simulink model "NeuronSizeActivity"  (Simulink 9.2)
settings: Solver=ode45  StartTime=0.0  StopTime=1  MaxStep=0.001  RelTol=1e-3  EnableMultiTasking=on
libraries: NeuroModelerLibrary x56
settings Model: Creator=Timba  LastModifiedBy=Bakhshiev  ExtModeTrigMode=oneshot  ExtModeArmWhenConnect=off
settings DataIOCC: LimitDataPoints=off
settings OptimizationCC: BlockReduction=off  BooleanDataType=off
settings DebuggingCC: SaveWithParameterizedLinksMsg=none  SignalResolutionControl=TryResolveAllWithWarning  MultiTaskDSMMsg=warning  MultiTaskCondExecSysMsg=none  FcnCallInpInsideContextMsg=error  StateNameClashWarn=none
settings HardwareCC: TargetUnknown=on
settings GRTTargetCC: TargetFcnLib=ansi_tfl_tmw.mat
settings ConfigComp: CovSFcnEnable=off

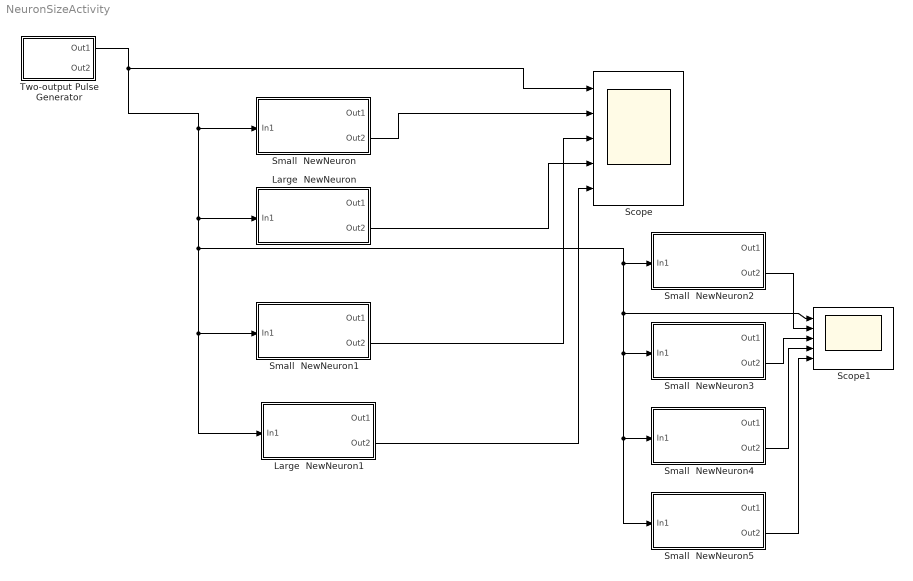
== system NeuronSizeActivity ==
  Large  NewNeuron : Subsystem
  Large  NewNeuron1 : Subsystem
  Scope : Scope  NumInputPorts=5
  Scope1 : Scope  NumInputPorts=5
  Small  NewNeuron : Subsystem
  Small  NewNeuron1 : Subsystem
  Small  NewNeuron2 : Subsystem
  Small  NewNeuron3 : Subsystem
  Small  NewNeuron4 : Subsystem
  Small  NewNeuron5 : Subsystem
  Two-output Pulse Generator : Subsystem  mask{A=100, P1=400, P2=100, PW=1, ST=0.001, OOn1=0.04, OOff1=0.5, OOn2=0.4, OOff2=20}
      mask prompts: A "Amplitude"; P1 "Out1: Period (number of samples)"; P2 "Out2: Period (number of samples)"; PW "Pulse Width (number of samples)"; ST "Sample Time"; OOn1 "Out1 On (seconds)"; OOff1 "Out1 Off (seconds)"; OOn2 "Out2 On (seconds)"; OOff2 "Out2 Off (seconds)"
  wires:
  Two-output Pulse Generator/1(Out1) -> Small  NewNeuron/1(In1), Large  NewNeuron/1(In1), Small  NewNeuron1/1(In1), Large  NewNeuron1/1(In1), Small  NewNeuron2/1(In1), Small  NewNeuron3/1(In1), Small  NewNeuron4/1(In1), Small  NewNeuron5/1(In1), Scope1/1, Scope/1
  Small  NewNeuron/2(Out2) -> Scope/2
  Small  NewNeuron1/2(Out2) -> Scope/3
  Large  NewNeuron1/2(Out2) -> Scope/5
  Large  NewNeuron/2(Out2) -> Scope/4
  Small  NewNeuron2/2(Out2) -> Scope1/2
  Small  NewNeuron3/2(Out2) -> Scope1/3
  Small  NewNeuron4/2(Out2) -> Scope1/4
  Small  NewNeuron5/2(Out2) -> Scope1/5

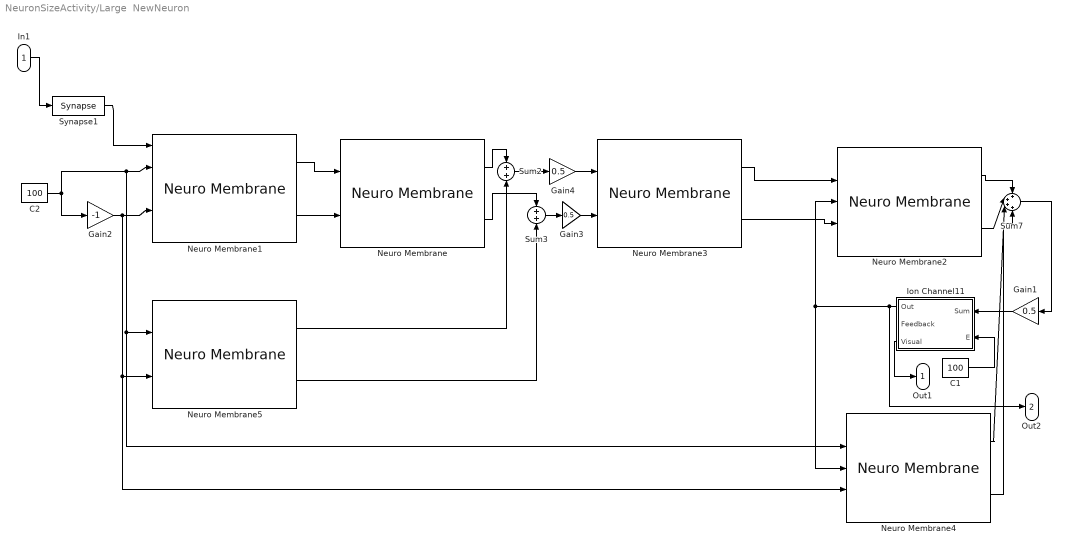
== system NeuronSizeActivity/Large  NewNeuron ==
  In1 : Inport
  C1 : Constant  Value=100
  C2 : Constant  Value=100
  Gain1 : Gain  Gain=0.5  OutDataTypeStr=Inherit: Same as input  ParamDataTypeStr=Inherit: Same as input
  Gain2 : Gain  Gain=-1  OutDataTypeStr=Inherit: Same as input  ParamDataTypeStr=Inherit: Same as input
  Gain3 : Gain  Gain=0.5  OutDataTypeStr=Inherit: Same as input  ParamDataTypeStr=Inherit: Same as input
  Gain4 : Gain  Gain=0.5  OutDataTypeStr=Inherit: Same as input  ParamDataTypeStr=Inherit: Same as input
  Ion Channel11 : Subsystem  mask(Ion pump){Rc=1, Cc=0.001, RR=1, IT=0.005, T=10}
      mask prompts: Rc "Channel resistance"; Cc "Channel capacity"; RR "Recharge Resistance"; IT "Input TC"; T "Threshold"
  Neuro Membrane{,1..5} (6 alike) : NeuroModelerLibrary/Old Neuron Elements/Neuro Membrane  ACm=0.1  ARm=1  ECm=0.1  ERm=1
  Sum2 : Sum  SaturateOnIntegerOverflow=on  InputSameDT=on  OutDataTypeStr=Inherit: Same as first input
  Sum3 : Sum  SaturateOnIntegerOverflow=on  InputSameDT=on  OutDataTypeStr=Inherit: Same as first input
  Sum7 : Sum  Inputs=++++  SaturateOnIntegerOverflow=on  InputSameDT=on  OutDataTypeStr=Inherit: Same as first input
  Synapse1 : NeuroModelerLibrary/Old Neuron Elements/Synapse  SecretionTC=0.001  DecompositionTC=0.1  ksi=1  gamma=1
  Out1 : Outport
  Out2 : Outport  Port=2
  wires:
  C2/1 -> Neuro Membrane1/2, Neuro Membrane4/2, Neuro Membrane5/2, Gain2/1
  Gain2/1 -> Neuro Membrane1/4, Neuro Membrane4/4, Neuro Membrane5/4
  Neuro Membrane2/2 -> Sum7/2
  Sum7/1 -> Gain1/1
  Neuro Membrane2/1 -> Sum7/1
  C1/1 -> Ion Channel11/2(E)
  In1/1 -> Synapse1/1
  Synapse1/1 -> Neuro Membrane1/1
  Ion Channel11/1(Out) -> Out2/1, Neuro Membrane4/3, Neuro Membrane2/3
  Neuro Membrane1/1 -> Neuro Membrane/2
  Neuro Membrane1/2 -> Neuro Membrane/4
  Neuro Membrane3/1 -> Neuro Membrane2/2
  Neuro Membrane3/2 -> Neuro Membrane2/4
  Neuro Membrane/1 -> Sum2/1
  Neuro Membrane/2 -> Sum3/1
  Sum3/1 -> Gain3/1
  Sum2/1 -> Gain4/1
  Neuro Membrane5/1 -> Sum2/2
  Neuro Membrane5/2 -> Sum3/2
  Gain1/1 -> Ion Channel11/1(Sum)
  Ion Channel11/3(Visual) -> Out1/1
  Gain3/1 -> Neuro Membrane3/4
  Gain4/1 -> Neuro Membrane3/2
  Neuro Membrane4/1 -> Sum7/3
  Neuro Membrane4/2 -> Sum7/4

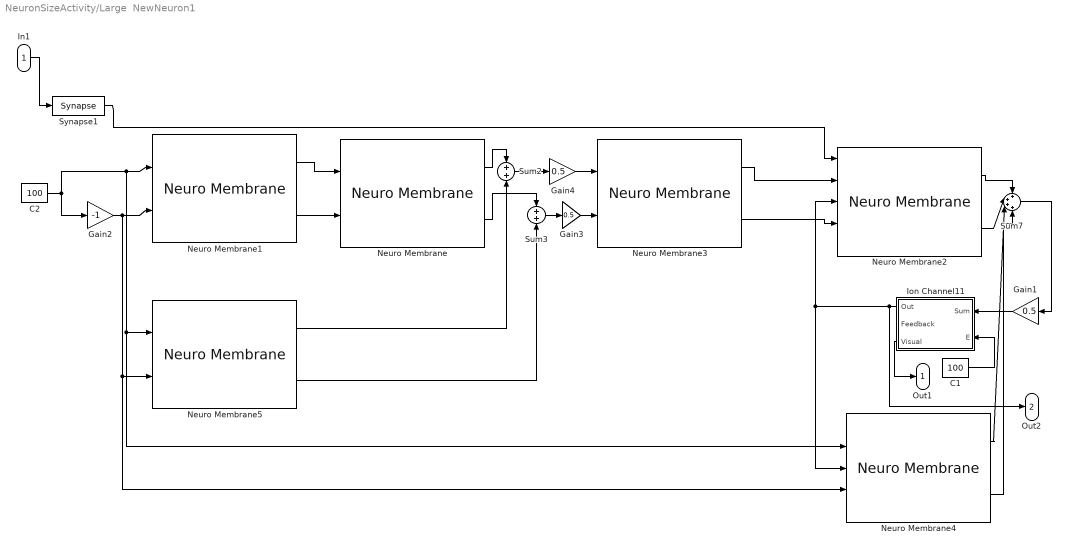
== system NeuronSizeActivity/Large  NewNeuron1 ==
  In1 : Inport
  C1 : Constant  Value=100
  C2 : Constant  Value=100
  Gain1 : Gain  Gain=0.5  OutDataTypeStr=Inherit: Same as input  ParamDataTypeStr=Inherit: Same as input
  Gain2 : Gain  Gain=-1  OutDataTypeStr=Inherit: Same as input  ParamDataTypeStr=Inherit: Same as input
  Gain3 : Gain  Gain=0.5  OutDataTypeStr=Inherit: Same as input  ParamDataTypeStr=Inherit: Same as input
  Gain4 : Gain  Gain=0.5  OutDataTypeStr=Inherit: Same as input  ParamDataTypeStr=Inherit: Same as input
  Ion Channel11 : Subsystem  mask(Ion pump){Rc=1, Cc=0.001, RR=1, IT=0.005, T=10}
      mask prompts: Rc "Channel resistance"; Cc "Channel capacity"; RR "Recharge Resistance"; IT "Input TC"; T "Threshold"
  Neuro Membrane{,1..5} (6 alike) : NeuroModelerLibrary/Old Neuron Elements/Neuro Membrane  ACm=0.1  ARm=1  ECm=0.1  ERm=1
  Sum2 : Sum  SaturateOnIntegerOverflow=on  InputSameDT=on  OutDataTypeStr=Inherit: Same as first input
  Sum3 : Sum  SaturateOnIntegerOverflow=on  InputSameDT=on  OutDataTypeStr=Inherit: Same as first input
  Sum7 : Sum  Inputs=++++  SaturateOnIntegerOverflow=on  InputSameDT=on  OutDataTypeStr=Inherit: Same as first input
  Synapse1 : NeuroModelerLibrary/Old Neuron Elements/Synapse  SecretionTC=0.001  DecompositionTC=0.1  ksi=1  gamma=1
  Out1 : Outport
  Out2 : Outport  Port=2
  wires:
  C2/1 -> Neuro Membrane1/2, Neuro Membrane4/2, Neuro Membrane5/2, Gain2/1
  Gain2/1 -> Neuro Membrane1/4, Neuro Membrane4/4, Neuro Membrane5/4
  Neuro Membrane2/2 -> Sum7/2
  Sum7/1 -> Gain1/1
  Neuro Membrane2/1 -> Sum7/1
  C1/1 -> Ion Channel11/2(E)
  In1/1 -> Synapse1/1
  Synapse1/1 -> Neuro Membrane2/1
  Ion Channel11/1(Out) -> Out2/1, Neuro Membrane4/3, Neuro Membrane2/3
  Neuro Membrane1/1 -> Neuro Membrane/2
  Neuro Membrane1/2 -> Neuro Membrane/4
  Neuro Membrane3/1 -> Neuro Membrane2/2
  Neuro Membrane3/2 -> Neuro Membrane2/4
  Neuro Membrane/1 -> Sum2/1
  Neuro Membrane/2 -> Sum3/1
  Sum3/1 -> Gain3/1
  Sum2/1 -> Gain4/1
  Neuro Membrane5/1 -> Sum2/2
  Neuro Membrane5/2 -> Sum3/2
  Gain1/1 -> Ion Channel11/1(Sum)
  Ion Channel11/3(Visual) -> Out1/1
  Gain3/1 -> Neuro Membrane3/4
  Gain4/1 -> Neuro Membrane3/2
  Neuro Membrane4/1 -> Sum7/3
  Neuro Membrane4/2 -> Sum7/4

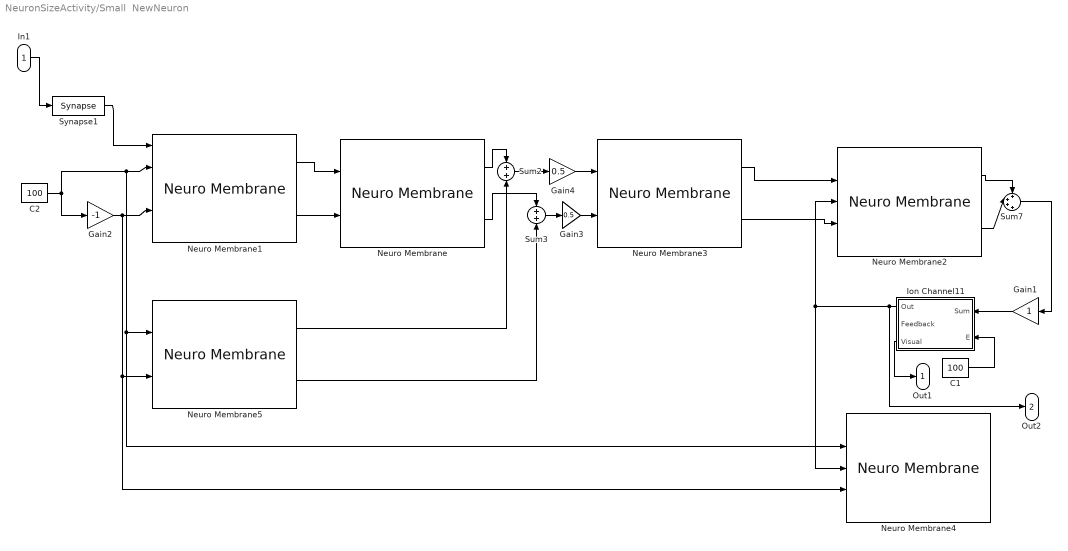
== system NeuronSizeActivity/Small  NewNeuron ==
  In1 : Inport
  C1 : Constant  Value=100
  C2 : Constant  Value=100
  Gain1 : Gain  OutDataTypeStr=Inherit: Same as input  ParamDataTypeStr=Inherit: Same as input
  Gain2 : Gain  Gain=-1  OutDataTypeStr=Inherit: Same as input  ParamDataTypeStr=Inherit: Same as input
  Gain3 : Gain  Gain=0.5  OutDataTypeStr=Inherit: Same as input  ParamDataTypeStr=Inherit: Same as input
  Gain4 : Gain  Gain=0.5  OutDataTypeStr=Inherit: Same as input  ParamDataTypeStr=Inherit: Same as input
  Ion Channel11 : Subsystem  mask(Ion pump){Rc=1, Cc=0.001, RR=1, IT=0.005, T=10}
      mask prompts: Rc "Channel resistance"; Cc "Channel capacity"; RR "Recharge Resistance"; IT "Input TC"; T "Threshold"
  Neuro Membrane{,1..5} (6 alike) : NeuroModelerLibrary/Old Neuron Elements/Neuro Membrane  ACm=0.1  ARm=1  ECm=0.1  ERm=1
  Sum2 : Sum  SaturateOnIntegerOverflow=on  InputSameDT=on  OutDataTypeStr=Inherit: Same as first input
  Sum3 : Sum  SaturateOnIntegerOverflow=on  InputSameDT=on  OutDataTypeStr=Inherit: Same as first input
  Sum7 : Sum  Inputs=++++  SaturateOnIntegerOverflow=on  InputSameDT=on  OutDataTypeStr=Inherit: Same as first input
  Synapse1 : NeuroModelerLibrary/Old Neuron Elements/Synapse  SecretionTC=0.001  DecompositionTC=0.1  ksi=1  gamma=1
  Out1 : Outport
  Out2 : Outport  Port=2
  wires:
  C2/1 -> Neuro Membrane1/2, Neuro Membrane4/2, Neuro Membrane5/2, Gain2/1
  Gain2/1 -> Neuro Membrane1/4, Neuro Membrane4/4, Neuro Membrane5/4
  Neuro Membrane2/2 -> Sum7/2
  Sum7/1 -> Gain1/1
  Neuro Membrane2/1 -> Sum7/1
  C1/1 -> Ion Channel11/2(E)
  In1/1 -> Synapse1/1
  Synapse1/1 -> Neuro Membrane1/1
  Ion Channel11/1(Out) -> Out2/1, Neuro Membrane4/3, Neuro Membrane2/3
  Neuro Membrane1/1 -> Neuro Membrane/2
  Neuro Membrane1/2 -> Neuro Membrane/4
  Neuro Membrane3/1 -> Neuro Membrane2/2
  Neuro Membrane3/2 -> Neuro Membrane2/4
  Neuro Membrane/1 -> Sum2/1
  Neuro Membrane/2 -> Sum3/1
  Sum3/1 -> Gain3/1
  Sum2/1 -> Gain4/1
  Neuro Membrane5/1 -> Sum2/2
  Neuro Membrane5/2 -> Sum3/2
  Gain1/1 -> Ion Channel11/1(Sum)
  Ion Channel11/3(Visual) -> Out1/1
  Gain3/1 -> Neuro Membrane3/4
  Gain4/1 -> Neuro Membrane3/2

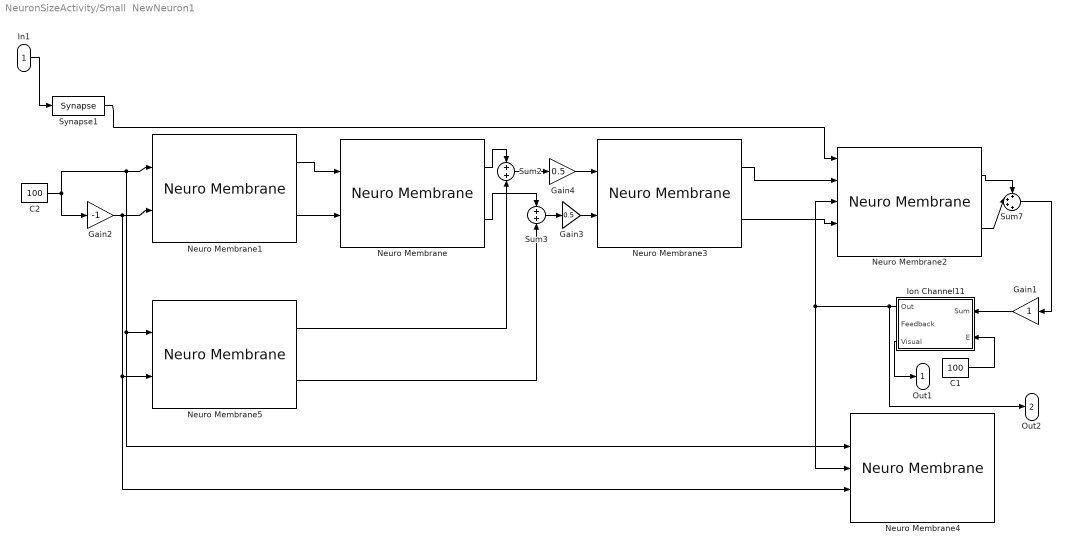
== system NeuronSizeActivity/Small  NewNeuron1 ==
  In1 : Inport
  C1 : Constant  Value=100
  C2 : Constant  Value=100
  Gain1 : Gain  OutDataTypeStr=Inherit: Same as input  ParamDataTypeStr=Inherit: Same as input
  Gain2 : Gain  Gain=-1  OutDataTypeStr=Inherit: Same as input  ParamDataTypeStr=Inherit: Same as input
  Gain3 : Gain  Gain=0.5  OutDataTypeStr=Inherit: Same as input  ParamDataTypeStr=Inherit: Same as input
  Gain4 : Gain  Gain=0.5  OutDataTypeStr=Inherit: Same as input  ParamDataTypeStr=Inherit: Same as input
  Ion Channel11 : Subsystem  mask(Ion pump){Rc=1, Cc=0.001, RR=1, IT=0.005, T=10}
      mask prompts: Rc "Channel resistance"; Cc "Channel capacity"; RR "Recharge Resistance"; IT "Input TC"; T "Threshold"
  Neuro Membrane{,1..5} (6 alike) : NeuroModelerLibrary/Old Neuron Elements/Neuro Membrane  ACm=0.1  ARm=1  ECm=0.1  ERm=1
  Sum2 : Sum  SaturateOnIntegerOverflow=on  InputSameDT=on  OutDataTypeStr=Inherit: Same as first input
  Sum3 : Sum  SaturateOnIntegerOverflow=on  InputSameDT=on  OutDataTypeStr=Inherit: Same as first input
  Sum7 : Sum  Inputs=++++  SaturateOnIntegerOverflow=on  InputSameDT=on  OutDataTypeStr=Inherit: Same as first input
  Synapse1 : NeuroModelerLibrary/Old Neuron Elements/Synapse  SecretionTC=0.001  DecompositionTC=0.1  ksi=1  gamma=1
  Out1 : Outport
  Out2 : Outport  Port=2
  wires:
  C2/1 -> Neuro Membrane1/2, Neuro Membrane4/2, Neuro Membrane5/2, Gain2/1
  Gain2/1 -> Neuro Membrane1/4, Neuro Membrane4/4, Neuro Membrane5/4
  Neuro Membrane2/2 -> Sum7/2
  Sum7/1 -> Gain1/1
  Neuro Membrane2/1 -> Sum7/1
  C1/1 -> Ion Channel11/2(E)
  In1/1 -> Synapse1/1
  Synapse1/1 -> Neuro Membrane2/1
  Ion Channel11/1(Out) -> Out2/1, Neuro Membrane4/3, Neuro Membrane2/3
  Neuro Membrane1/1 -> Neuro Membrane/2
  Neuro Membrane1/2 -> Neuro Membrane/4
  Neuro Membrane3/1 -> Neuro Membrane2/2
  Neuro Membrane3/2 -> Neuro Membrane2/4
  Neuro Membrane/1 -> Sum2/1
  Neuro Membrane/2 -> Sum3/1
  Sum3/1 -> Gain3/1
  Sum2/1 -> Gain4/1
  Neuro Membrane5/1 -> Sum2/2
  Neuro Membrane5/2 -> Sum3/2
  Gain1/1 -> Ion Channel11/1(Sum)
  Ion Channel11/3(Visual) -> Out1/1
  Gain3/1 -> Neuro Membrane3/4
  Gain4/1 -> Neuro Membrane3/2

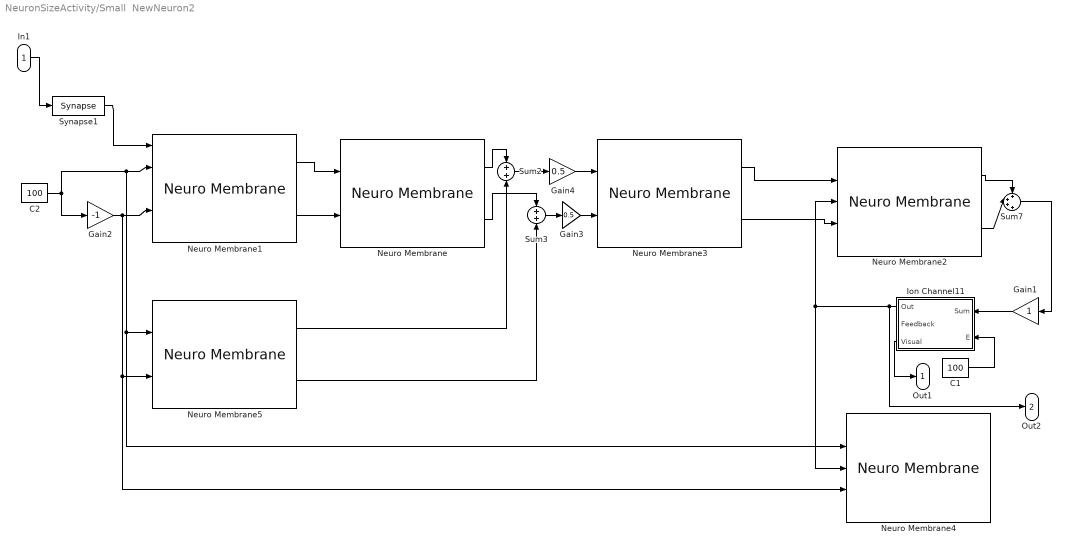
== system NeuronSizeActivity/Small  NewNeuron2 ==
  In1 : Inport
  C1 : Constant  Value=100
  C2 : Constant  Value=100
  Gain1 : Gain  OutDataTypeStr=Inherit: Same as input  ParamDataTypeStr=Inherit: Same as input
  Gain2 : Gain  Gain=-1  OutDataTypeStr=Inherit: Same as input  ParamDataTypeStr=Inherit: Same as input
  Gain3 : Gain  Gain=0.5  OutDataTypeStr=Inherit: Same as input  ParamDataTypeStr=Inherit: Same as input
  Gain4 : Gain  Gain=0.5  OutDataTypeStr=Inherit: Same as input  ParamDataTypeStr=Inherit: Same as input
  Ion Channel11 : Subsystem  mask(Ion pump){Rc=1, Cc=0.001, RR=1, IT=0.005, T=10}
      mask prompts: Rc "Channel resistance"; Cc "Channel capacity"; RR "Recharge Resistance"; IT "Input TC"; T "Threshold"
  Neuro Membrane{,1..5} (6 alike) : NeuroModelerLibrary/Old Neuron Elements/Neuro Membrane  ACm=0.1  ARm=1  ECm=0.1  ERm=1
  Sum2 : Sum  SaturateOnIntegerOverflow=on  InputSameDT=on  OutDataTypeStr=Inherit: Same as first input
  Sum3 : Sum  SaturateOnIntegerOverflow=on  InputSameDT=on  OutDataTypeStr=Inherit: Same as first input
  Sum7 : Sum  Inputs=++++  SaturateOnIntegerOverflow=on  InputSameDT=on  OutDataTypeStr=Inherit: Same as first input
  Synapse1 : NeuroModelerLibrary/Old Neuron Elements/Synapse  SecretionTC=0.001  DecompositionTC=0.1  ksi=1  gamma=1
  Out1 : Outport
  Out2 : Outport  Port=2
  wires:
  C2/1 -> Neuro Membrane1/2, Neuro Membrane4/2, Neuro Membrane5/2, Gain2/1
  Gain2/1 -> Neuro Membrane1/4, Neuro Membrane4/4, Neuro Membrane5/4
  Neuro Membrane2/2 -> Sum7/2
  Sum7/1 -> Gain1/1
  Neuro Membrane2/1 -> Sum7/1
  C1/1 -> Ion Channel11/2(E)
  In1/1 -> Synapse1/1
  Synapse1/1 -> Neuro Membrane1/1
  Ion Channel11/1(Out) -> Out2/1, Neuro Membrane4/3, Neuro Membrane2/3
  Neuro Membrane1/1 -> Neuro Membrane/2
  Neuro Membrane1/2 -> Neuro Membrane/4
  Neuro Membrane3/1 -> Neuro Membrane2/2
  Neuro Membrane3/2 -> Neuro Membrane2/4
  Neuro Membrane/1 -> Sum2/1
  Neuro Membrane/2 -> Sum3/1
  Sum3/1 -> Gain3/1
  Sum2/1 -> Gain4/1
  Neuro Membrane5/1 -> Sum2/2
  Neuro Membrane5/2 -> Sum3/2
  Gain1/1 -> Ion Channel11/1(Sum)
  Ion Channel11/3(Visual) -> Out1/1
  Gain3/1 -> Neuro Membrane3/4
  Gain4/1 -> Neuro Membrane3/2

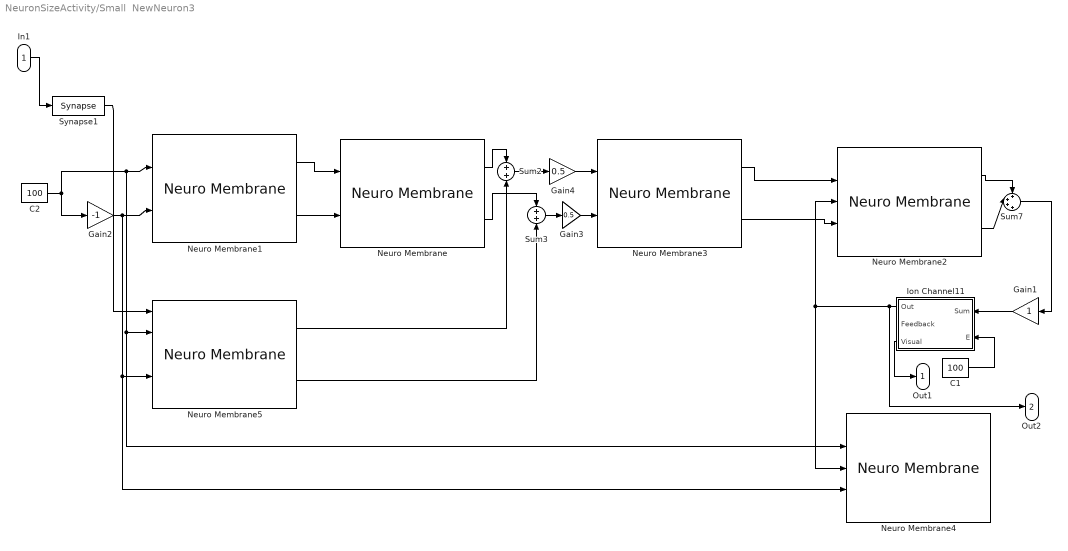
== system NeuronSizeActivity/Small  NewNeuron3 ==
  In1 : Inport
  C1 : Constant  Value=100
  C2 : Constant  Value=100
  Gain1 : Gain  OutDataTypeStr=Inherit: Same as input  ParamDataTypeStr=Inherit: Same as input
  Gain2 : Gain  Gain=-1  OutDataTypeStr=Inherit: Same as input  ParamDataTypeStr=Inherit: Same as input
  Gain3 : Gain  Gain=0.5  OutDataTypeStr=Inherit: Same as input  ParamDataTypeStr=Inherit: Same as input
  Gain4 : Gain  Gain=0.5  OutDataTypeStr=Inherit: Same as input  ParamDataTypeStr=Inherit: Same as input
  Ion Channel11 : Subsystem  mask(Ion pump){Rc=1, Cc=0.001, RR=1, IT=0.005, T=10}
      mask prompts: Rc "Channel resistance"; Cc "Channel capacity"; RR "Recharge Resistance"; IT "Input TC"; T "Threshold"
  Neuro Membrane{,1..5} (6 alike) : NeuroModelerLibrary/Old Neuron Elements/Neuro Membrane  ACm=0.1  ARm=1  ECm=0.1  ERm=1
  Sum2 : Sum  SaturateOnIntegerOverflow=on  InputSameDT=on  OutDataTypeStr=Inherit: Same as first input
  Sum3 : Sum  SaturateOnIntegerOverflow=on  InputSameDT=on  OutDataTypeStr=Inherit: Same as first input
  Sum7 : Sum  Inputs=++++  SaturateOnIntegerOverflow=on  InputSameDT=on  OutDataTypeStr=Inherit: Same as first input
  Synapse1 : NeuroModelerLibrary/Old Neuron Elements/Synapse  SecretionTC=0.001  DecompositionTC=0.1  ksi=1  gamma=1
  Out1 : Outport
  Out2 : Outport  Port=2
  wires:
  C2/1 -> Neuro Membrane1/2, Neuro Membrane4/2, Neuro Membrane5/2, Gain2/1
  Gain2/1 -> Neuro Membrane1/4, Neuro Membrane4/4, Neuro Membrane5/4
  Neuro Membrane2/2 -> Sum7/2
  Sum7/1 -> Gain1/1
  Neuro Membrane2/1 -> Sum7/1
  C1/1 -> Ion Channel11/2(E)
  In1/1 -> Synapse1/1
  Synapse1/1 -> Neuro Membrane5/1
  Ion Channel11/1(Out) -> Out2/1, Neuro Membrane4/3, Neuro Membrane2/3
  Neuro Membrane1/1 -> Neuro Membrane/2
  Neuro Membrane1/2 -> Neuro Membrane/4
  Neuro Membrane3/1 -> Neuro Membrane2/2
  Neuro Membrane3/2 -> Neuro Membrane2/4
  Neuro Membrane/1 -> Sum2/1
  Neuro Membrane/2 -> Sum3/1
  Sum3/1 -> Gain3/1
  Sum2/1 -> Gain4/1
  Neuro Membrane5/1 -> Sum2/2
  Neuro Membrane5/2 -> Sum3/2
  Gain1/1 -> Ion Channel11/1(Sum)
  Ion Channel11/3(Visual) -> Out1/1
  Gain3/1 -> Neuro Membrane3/4
  Gain4/1 -> Neuro Membrane3/2

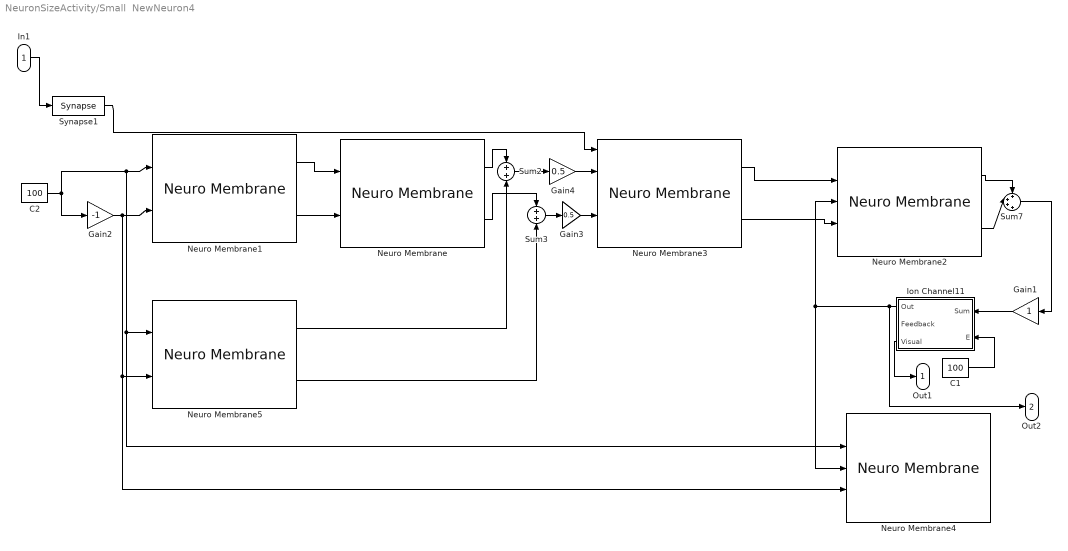
== system NeuronSizeActivity/Small  NewNeuron4 ==
  In1 : Inport
  C1 : Constant  Value=100
  C2 : Constant  Value=100
  Gain1 : Gain  OutDataTypeStr=Inherit: Same as input  ParamDataTypeStr=Inherit: Same as input
  Gain2 : Gain  Gain=-1  OutDataTypeStr=Inherit: Same as input  ParamDataTypeStr=Inherit: Same as input
  Gain3 : Gain  Gain=0.5  OutDataTypeStr=Inherit: Same as input  ParamDataTypeStr=Inherit: Same as input
  Gain4 : Gain  Gain=0.5  OutDataTypeStr=Inherit: Same as input  ParamDataTypeStr=Inherit: Same as input
  Ion Channel11 : Subsystem  mask(Ion pump){Rc=1, Cc=0.001, RR=1, IT=0.005, T=10}
      mask prompts: Rc "Channel resistance"; Cc "Channel capacity"; RR "Recharge Resistance"; IT "Input TC"; T "Threshold"
  Neuro Membrane{,1..5} (6 alike) : NeuroModelerLibrary/Old Neuron Elements/Neuro Membrane  ACm=0.1  ARm=1  ECm=0.1  ERm=1
  Sum2 : Sum  SaturateOnIntegerOverflow=on  InputSameDT=on  OutDataTypeStr=Inherit: Same as first input
  Sum3 : Sum  SaturateOnIntegerOverflow=on  InputSameDT=on  OutDataTypeStr=Inherit: Same as first input
  Sum7 : Sum  Inputs=++++  SaturateOnIntegerOverflow=on  InputSameDT=on  OutDataTypeStr=Inherit: Same as first input
  Synapse1 : NeuroModelerLibrary/Old Neuron Elements/Synapse  SecretionTC=0.001  DecompositionTC=0.1  ksi=1  gamma=1
  Out1 : Outport
  Out2 : Outport  Port=2
  wires:
  C2/1 -> Neuro Membrane1/2, Neuro Membrane4/2, Neuro Membrane5/2, Gain2/1
  Gain2/1 -> Neuro Membrane1/4, Neuro Membrane4/4, Neuro Membrane5/4
  Neuro Membrane2/2 -> Sum7/2
  Sum7/1 -> Gain1/1
  Neuro Membrane2/1 -> Sum7/1
  C1/1 -> Ion Channel11/2(E)
  In1/1 -> Synapse1/1
  Synapse1/1 -> Neuro Membrane3/1
  Ion Channel11/1(Out) -> Out2/1, Neuro Membrane4/3, Neuro Membrane2/3
  Neuro Membrane1/1 -> Neuro Membrane/2
  Neuro Membrane1/2 -> Neuro Membrane/4
  Neuro Membrane3/1 -> Neuro Membrane2/2
  Neuro Membrane3/2 -> Neuro Membrane2/4
  Neuro Membrane/1 -> Sum2/1
  Neuro Membrane/2 -> Sum3/1
  Sum3/1 -> Gain3/1
  Sum2/1 -> Gain4/1
  Neuro Membrane5/1 -> Sum2/2
  Neuro Membrane5/2 -> Sum3/2
  Gain1/1 -> Ion Channel11/1(Sum)
  Ion Channel11/3(Visual) -> Out1/1
  Gain3/1 -> Neuro Membrane3/4
  Gain4/1 -> Neuro Membrane3/2

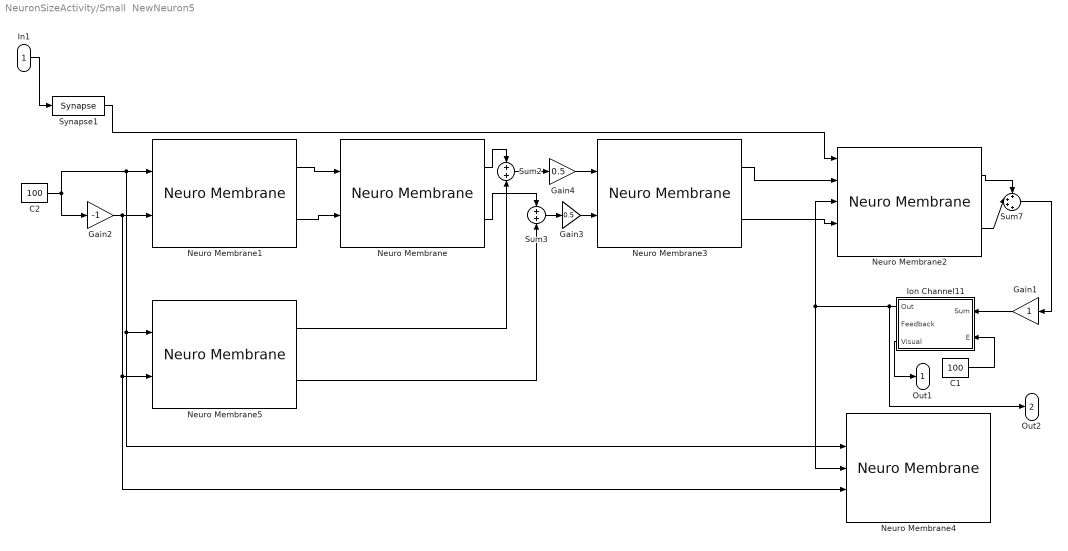
== system NeuronSizeActivity/Small  NewNeuron5 ==
  In1 : Inport
  C1 : Constant  Value=100
  C2 : Constant  Value=100
  Gain1 : Gain  OutDataTypeStr=Inherit: Same as input  ParamDataTypeStr=Inherit: Same as input
  Gain2 : Gain  Gain=-1  OutDataTypeStr=Inherit: Same as input  ParamDataTypeStr=Inherit: Same as input
  Gain3 : Gain  Gain=0.5  OutDataTypeStr=Inherit: Same as input  ParamDataTypeStr=Inherit: Same as input
  Gain4 : Gain  Gain=0.5  OutDataTypeStr=Inherit: Same as input  ParamDataTypeStr=Inherit: Same as input
  Ion Channel11 : Subsystem  mask(Ion pump){Rc=1, Cc=0.001, RR=1, IT=0.005, T=10}
      mask prompts: Rc "Channel resistance"; Cc "Channel capacity"; RR "Recharge Resistance"; IT "Input TC"; T "Threshold"
  Neuro Membrane{,1..5} (6 alike) : NeuroModelerLibrary/Old Neuron Elements/Neuro Membrane  ACm=0.1  ARm=1  ECm=0.1  ERm=1
  Sum2 : Sum  SaturateOnIntegerOverflow=on  InputSameDT=on  OutDataTypeStr=Inherit: Same as first input
  Sum3 : Sum  SaturateOnIntegerOverflow=on  InputSameDT=on  OutDataTypeStr=Inherit: Same as first input
  Sum7 : Sum  Inputs=++++  SaturateOnIntegerOverflow=on  InputSameDT=on  OutDataTypeStr=Inherit: Same as first input
  Synapse1 : NeuroModelerLibrary/Old Neuron Elements/Synapse  SecretionTC=0.001  DecompositionTC=0.1  ksi=1  gamma=1
  Out1 : Outport
  Out2 : Outport  Port=2
  wires:
  C2/1 -> Neuro Membrane1/2, Neuro Membrane4/2, Neuro Membrane5/2, Gain2/1
  Gain2/1 -> Neuro Membrane1/4, Neuro Membrane4/4, Neuro Membrane5/4
  Neuro Membrane2/2 -> Sum7/2
  Sum7/1 -> Gain1/1
  Neuro Membrane2/1 -> Sum7/1
  C1/1 -> Ion Channel11/2(E)
  In1/1 -> Synapse1/1
  Synapse1/1 -> Neuro Membrane2/1
  Ion Channel11/1(Out) -> Out2/1, Neuro Membrane4/3, Neuro Membrane2/3
  Neuro Membrane1/1 -> Neuro Membrane/2
  Neuro Membrane1/2 -> Neuro Membrane/4
  Neuro Membrane3/1 -> Neuro Membrane2/2
  Neuro Membrane3/2 -> Neuro Membrane2/4
  Neuro Membrane/1 -> Sum2/1
  Neuro Membrane/2 -> Sum3/1
  Sum3/1 -> Gain3/1
  Sum2/1 -> Gain4/1
  Neuro Membrane5/1 -> Sum2/2
  Neuro Membrane5/2 -> Sum3/2
  Gain1/1 -> Ion Channel11/1(Sum)
  Ion Channel11/3(Visual) -> Out1/1
  Gain3/1 -> Neuro Membrane3/4
  Gain4/1 -> Neuro Membrane3/2

== system NeuronSizeActivity/Two-output Pulse Generator ==
  Clock : Clock
  Constant : Constant  Value=0
  Discrete Pulse Generator : DiscretePulseGenerator  Amplitude=A  Period=P1  PulseWidth=PW  SampleTime=ST
  Discrete Pulse Generator1 : DiscretePulseGenerator  Amplitude=A  Period=P2  PulseWidth=PW  SampleTime=ST
  Switch : Switch  Threshold=OOff1  SaturateOnIntegerOverflow=on  InputSameDT=on
  Switch1 : Switch  Threshold=OOff2  SaturateOnIntegerOverflow=on  InputSameDT=on
  Transport Delay : TransportDelay  DelayTime=OOn1
  Transport Delay1 : TransportDelay  DelayTime=OOn2
  Out1 : Outport  InitialOutput=0
  Out2 : Outport  Port=2  InitialOutput=0
  wires:
  Discrete Pulse Generator/1 -> Transport Delay/1
  Constant/1 -> Switch/1, Switch1/1
  Discrete Pulse Generator1/1 -> Transport Delay1/1
  Transport Delay1/1 -> Switch1/3
  Transport Delay/1 -> Switch/3
  Clock/1 -> Switch/2, Switch1/2
  Switch/1 -> Out1/1
  Switch1/1 -> Out2/1

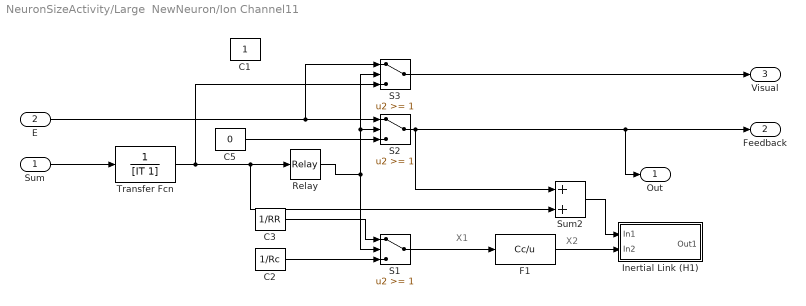
== system NeuronSizeActivity/Large  NewNeuron/Ion Channel11 ==
  note: X2
  note: X1
  Sum : Inport
  E : Inport  Port=2
  C1 : Constant
  C2 : Constant  Value=1/Rc
  C3 : Constant  Value=1/RR
  C5 : Constant  Value=0
  F1 : Fcn  Expr=Cc/u
  Inertial Link (H1) : Subsystem
  Relay : Relay  OnSwitchValue=T  OffSwitchValue=0
  S1 : Switch  Threshold=1  SaturateOnIntegerOverflow=on  InputSameDT=on
  S2 : Switch  Threshold=1  SaturateOnIntegerOverflow=on  InputSameDT=on
  S3 : Switch  Threshold=1  SaturateOnIntegerOverflow=on  InputSameDT=on
  Sum2 : Sum  SaturateOnIntegerOverflow=on  InputSameDT=on  OutDataTypeStr=Inherit: Same as first input
  Transfer Fcn : TransferFcn  Denominator=[IT 1]
  Out : Outport  InitialOutput=0
  Feedback : Outport  Port=2  InitialOutput=0
  Visual : Outport  Port=3  InitialOutput=0
  wires:
  Sum2/1 -> Inertial Link (H1)/1(In1)
  F1/1 -> Inertial Link (H1)/2(In2)
  C2/1 -> S1/3
  C3/1 -> S1/1
  Sum/1 -> Transfer Fcn/1
  C5/1 -> S2/3
  E/1 -> S2/1, S3/1
  S2/1 -> Sum2/1, Feedback/1, Out/1
  S1/1 -> F1/1
  Transfer Fcn/1 -> Sum2/2, Relay/1, S3/3
  Relay/1 -> S1/2, S2/2, S3/2
  S3/1 -> Visual/1

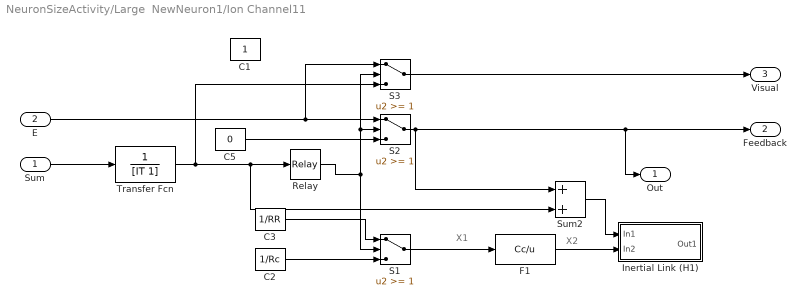
== system NeuronSizeActivity/Large  NewNeuron1/Ion Channel11 ==
  note: X2
  note: X1
  Sum : Inport
  E : Inport  Port=2
  C1 : Constant
  C2 : Constant  Value=1/Rc
  C3 : Constant  Value=1/RR
  C5 : Constant  Value=0
  F1 : Fcn  Expr=Cc/u
  Inertial Link (H1) : Subsystem
  Relay : Relay  OnSwitchValue=T  OffSwitchValue=0
  S1 : Switch  Threshold=1  SaturateOnIntegerOverflow=on  InputSameDT=on
  S2 : Switch  Threshold=1  SaturateOnIntegerOverflow=on  InputSameDT=on
  S3 : Switch  Threshold=1  SaturateOnIntegerOverflow=on  InputSameDT=on
  Sum2 : Sum  SaturateOnIntegerOverflow=on  InputSameDT=on  OutDataTypeStr=Inherit: Same as first input
  Transfer Fcn : TransferFcn  Denominator=[IT 1]
  Out : Outport  InitialOutput=0
  Feedback : Outport  Port=2  InitialOutput=0
  Visual : Outport  Port=3  InitialOutput=0
  wires:
  Sum2/1 -> Inertial Link (H1)/1(In1)
  F1/1 -> Inertial Link (H1)/2(In2)
  C2/1 -> S1/3
  C3/1 -> S1/1
  Sum/1 -> Transfer Fcn/1
  C5/1 -> S2/3
  E/1 -> S2/1, S3/1
  S2/1 -> Sum2/1, Feedback/1, Out/1
  S1/1 -> F1/1
  Transfer Fcn/1 -> Sum2/2, Relay/1, S3/3
  Relay/1 -> S1/2, S2/2, S3/2
  S3/1 -> Visual/1

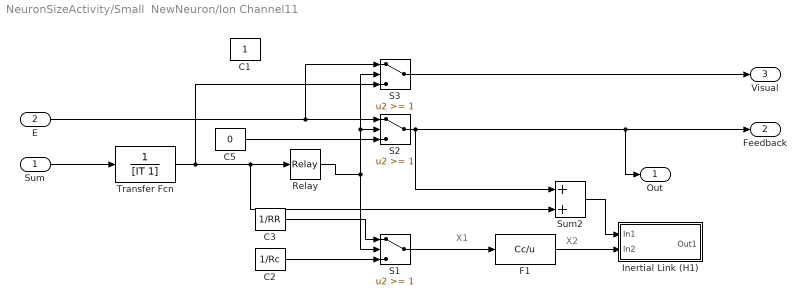
== system NeuronSizeActivity/Small  NewNeuron/Ion Channel11 ==
  note: X2
  note: X1
  Sum : Inport
  E : Inport  Port=2
  C1 : Constant
  C2 : Constant  Value=1/Rc
  C3 : Constant  Value=1/RR
  C5 : Constant  Value=0
  F1 : Fcn  Expr=Cc/u
  Inertial Link (H1) : Subsystem
  Relay : Relay  OnSwitchValue=T  OffSwitchValue=0
  S1 : Switch  Threshold=1  SaturateOnIntegerOverflow=on  InputSameDT=on
  S2 : Switch  Threshold=1  SaturateOnIntegerOverflow=on  InputSameDT=on
  S3 : Switch  Threshold=1  SaturateOnIntegerOverflow=on  InputSameDT=on
  Sum2 : Sum  SaturateOnIntegerOverflow=on  InputSameDT=on  OutDataTypeStr=Inherit: Same as first input
  Transfer Fcn : TransferFcn  Denominator=[IT 1]
  Out : Outport  InitialOutput=0
  Feedback : Outport  Port=2  InitialOutput=0
  Visual : Outport  Port=3  InitialOutput=0
  wires:
  Sum2/1 -> Inertial Link (H1)/1(In1)
  F1/1 -> Inertial Link (H1)/2(In2)
  C2/1 -> S1/3
  C3/1 -> S1/1
  Sum/1 -> Transfer Fcn/1
  C5/1 -> S2/3
  E/1 -> S2/1, S3/1
  S2/1 -> Sum2/1, Feedback/1, Out/1
  S1/1 -> F1/1
  Transfer Fcn/1 -> Sum2/2, Relay/1, S3/3
  Relay/1 -> S1/2, S2/2, S3/2
  S3/1 -> Visual/1

== system NeuronSizeActivity/Small  NewNeuron1/Ion Channel11 ==
  note: X2
  note: X1
  Sum : Inport
  E : Inport  Port=2
  C1 : Constant
  C2 : Constant  Value=1/Rc
  C3 : Constant  Value=1/RR
  C5 : Constant  Value=0
  F1 : Fcn  Expr=Cc/u
  Inertial Link (H1) : Subsystem
  Relay : Relay  OnSwitchValue=T  OffSwitchValue=0
  S1 : Switch  Threshold=1  SaturateOnIntegerOverflow=on  InputSameDT=on
  S2 : Switch  Threshold=1  SaturateOnIntegerOverflow=on  InputSameDT=on
  S3 : Switch  Threshold=1  SaturateOnIntegerOverflow=on  InputSameDT=on
  Sum2 : Sum  SaturateOnIntegerOverflow=on  InputSameDT=on  OutDataTypeStr=Inherit: Same as first input
  Transfer Fcn : TransferFcn  Denominator=[IT 1]
  Out : Outport  InitialOutput=0
  Feedback : Outport  Port=2  InitialOutput=0
  Visual : Outport  Port=3  InitialOutput=0
  wires:
  Sum2/1 -> Inertial Link (H1)/1(In1)
  F1/1 -> Inertial Link (H1)/2(In2)
  C2/1 -> S1/3
  C3/1 -> S1/1
  Sum/1 -> Transfer Fcn/1
  C5/1 -> S2/3
  E/1 -> S2/1, S3/1
  S2/1 -> Sum2/1, Feedback/1, Out/1
  S1/1 -> F1/1
  Transfer Fcn/1 -> Sum2/2, Relay/1, S3/3
  Relay/1 -> S1/2, S2/2, S3/2
  S3/1 -> Visual/1

== system NeuronSizeActivity/Small  NewNeuron2/Ion Channel11 ==
  note: X2
  note: X1
  Sum : Inport
  E : Inport  Port=2
  C1 : Constant
  C2 : Constant  Value=1/Rc
  C3 : Constant  Value=1/RR
  C5 : Constant  Value=0
  F1 : Fcn  Expr=Cc/u
  Inertial Link (H1) : Subsystem
  Relay : Relay  OnSwitchValue=T  OffSwitchValue=0
  S1 : Switch  Threshold=1  SaturateOnIntegerOverflow=on  InputSameDT=on
  S2 : Switch  Threshold=1  SaturateOnIntegerOverflow=on  InputSameDT=on
  S3 : Switch  Threshold=1  SaturateOnIntegerOverflow=on  InputSameDT=on
  Sum2 : Sum  SaturateOnIntegerOverflow=on  InputSameDT=on  OutDataTypeStr=Inherit: Same as first input
  Transfer Fcn : TransferFcn  Denominator=[IT 1]
  Out : Outport  InitialOutput=0
  Feedback : Outport  Port=2  InitialOutput=0
  Visual : Outport  Port=3  InitialOutput=0
  wires:
  Sum2/1 -> Inertial Link (H1)/1(In1)
  F1/1 -> Inertial Link (H1)/2(In2)
  C2/1 -> S1/3
  C3/1 -> S1/1
  Sum/1 -> Transfer Fcn/1
  C5/1 -> S2/3
  E/1 -> S2/1, S3/1
  S2/1 -> Sum2/1, Feedback/1, Out/1
  S1/1 -> F1/1
  Transfer Fcn/1 -> Sum2/2, Relay/1, S3/3
  Relay/1 -> S1/2, S2/2, S3/2
  S3/1 -> Visual/1

== system NeuronSizeActivity/Small  NewNeuron3/Ion Channel11 ==
  note: X2
  note: X1
  Sum : Inport
  E : Inport  Port=2
  C1 : Constant
  C2 : Constant  Value=1/Rc
  C3 : Constant  Value=1/RR
  C5 : Constant  Value=0
  F1 : Fcn  Expr=Cc/u
  Inertial Link (H1) : Subsystem
  Relay : Relay  OnSwitchValue=T  OffSwitchValue=0
  S1 : Switch  Threshold=1  SaturateOnIntegerOverflow=on  InputSameDT=on
  S2 : Switch  Threshold=1  SaturateOnIntegerOverflow=on  InputSameDT=on
  S3 : Switch  Threshold=1  SaturateOnIntegerOverflow=on  InputSameDT=on
  Sum2 : Sum  SaturateOnIntegerOverflow=on  InputSameDT=on  OutDataTypeStr=Inherit: Same as first input
  Transfer Fcn : TransferFcn  Denominator=[IT 1]
  Out : Outport  InitialOutput=0
  Feedback : Outport  Port=2  InitialOutput=0
  Visual : Outport  Port=3  InitialOutput=0
  wires:
  Sum2/1 -> Inertial Link (H1)/1(In1)
  F1/1 -> Inertial Link (H1)/2(In2)
  C2/1 -> S1/3
  C3/1 -> S1/1
  Sum/1 -> Transfer Fcn/1
  C5/1 -> S2/3
  E/1 -> S2/1, S3/1
  S2/1 -> Sum2/1, Feedback/1, Out/1
  S1/1 -> F1/1
  Transfer Fcn/1 -> Sum2/2, Relay/1, S3/3
  Relay/1 -> S1/2, S2/2, S3/2
  S3/1 -> Visual/1

== system NeuronSizeActivity/Small  NewNeuron4/Ion Channel11 ==
  note: X2
  note: X1
  Sum : Inport
  E : Inport  Port=2
  C1 : Constant
  C2 : Constant  Value=1/Rc
  C3 : Constant  Value=1/RR
  C5 : Constant  Value=0
  F1 : Fcn  Expr=Cc/u
  Inertial Link (H1) : Subsystem
  Relay : Relay  OnSwitchValue=T  OffSwitchValue=0
  S1 : Switch  Threshold=1  SaturateOnIntegerOverflow=on  InputSameDT=on
  S2 : Switch  Threshold=1  SaturateOnIntegerOverflow=on  InputSameDT=on
  S3 : Switch  Threshold=1  SaturateOnIntegerOverflow=on  InputSameDT=on
  Sum2 : Sum  SaturateOnIntegerOverflow=on  InputSameDT=on  OutDataTypeStr=Inherit: Same as first input
  Transfer Fcn : TransferFcn  Denominator=[IT 1]
  Out : Outport  InitialOutput=0
  Feedback : Outport  Port=2  InitialOutput=0
  Visual : Outport  Port=3  InitialOutput=0
  wires:
  Sum2/1 -> Inertial Link (H1)/1(In1)
  F1/1 -> Inertial Link (H1)/2(In2)
  C2/1 -> S1/3
  C3/1 -> S1/1
  Sum/1 -> Transfer Fcn/1
  C5/1 -> S2/3
  E/1 -> S2/1, S3/1
  S2/1 -> Sum2/1, Feedback/1, Out/1
  S1/1 -> F1/1
  Transfer Fcn/1 -> Sum2/2, Relay/1, S3/3
  Relay/1 -> S1/2, S2/2, S3/2
  S3/1 -> Visual/1

== system NeuronSizeActivity/Small  NewNeuron5/Ion Channel11 ==
  note: X2
  note: X1
  Sum : Inport
  E : Inport  Port=2
  C1 : Constant
  C2 : Constant  Value=1/Rc
  C3 : Constant  Value=1/RR
  C5 : Constant  Value=0
  F1 : Fcn  Expr=Cc/u
  Inertial Link (H1) : Subsystem
  Relay : Relay  OnSwitchValue=T  OffSwitchValue=0
  S1 : Switch  Threshold=1  SaturateOnIntegerOverflow=on  InputSameDT=on
  S2 : Switch  Threshold=1  SaturateOnIntegerOverflow=on  InputSameDT=on
  S3 : Switch  Threshold=1  SaturateOnIntegerOverflow=on  InputSameDT=on
  Sum2 : Sum  SaturateOnIntegerOverflow=on  InputSameDT=on  OutDataTypeStr=Inherit: Same as first input
  Transfer Fcn : TransferFcn  Denominator=[IT 1]
  Out : Outport  InitialOutput=0
  Feedback : Outport  Port=2  InitialOutput=0
  Visual : Outport  Port=3  InitialOutput=0
  wires:
  Sum2/1 -> Inertial Link (H1)/1(In1)
  F1/1 -> Inertial Link (H1)/2(In2)
  C2/1 -> S1/3
  C3/1 -> S1/1
  Sum/1 -> Transfer Fcn/1
  C5/1 -> S2/3
  E/1 -> S2/1, S3/1
  S2/1 -> Sum2/1, Feedback/1, Out/1
  S1/1 -> F1/1
  Transfer Fcn/1 -> Sum2/2, Relay/1, S3/3
  Relay/1 -> S1/2, S2/2, S3/2
  S3/1 -> Visual/1

== system NeuronSizeActivity/Large  NewNeuron/Ion Channel11/Inertial Link (H1) ==
  In1 : Inport
  In2 : Inport  Port=2
  Fcn1 : Fcn  Expr=1/u
  Integrator : Integrator
  Product : Product  SaturateOnIntegerOverflow=on  RndMeth=Zero  InputSameDT=on  OutDataTypeStr=Inherit: Same as first input
  Product1 : Product  SaturateOnIntegerOverflow=on  RndMeth=Zero  InputSameDT=on  OutDataTypeStr=Inherit: Same as first input
  Sum : Sum  Inputs=+-  SaturateOnIntegerOverflow=on  InputSameDT=on  OutDataTypeStr=Inherit: Same as first input
  Out1 : Outport  InitialOutput=0
  wires:
  Sum/1 -> Integrator/1
  Product/1 -> Sum/2
  Product1/1 -> Sum/1
  Fcn1/1 -> Product/2, Product1/2
  Integrator/1 -> Product/1, Out1/1
  In1/1 -> Product1/1
  In2/1 -> Fcn1/1

== system NeuronSizeActivity/Large  NewNeuron1/Ion Channel11/Inertial Link (H1) ==
  In1 : Inport
  In2 : Inport  Port=2
  Fcn1 : Fcn  Expr=1/u
  Integrator : Integrator
  Product : Product  SaturateOnIntegerOverflow=on  RndMeth=Zero  InputSameDT=on  OutDataTypeStr=Inherit: Same as first input
  Product1 : Product  SaturateOnIntegerOverflow=on  RndMeth=Zero  InputSameDT=on  OutDataTypeStr=Inherit: Same as first input
  Sum : Sum  Inputs=+-  SaturateOnIntegerOverflow=on  InputSameDT=on  OutDataTypeStr=Inherit: Same as first input
  Out1 : Outport  InitialOutput=0
  wires:
  Sum/1 -> Integrator/1
  Product/1 -> Sum/2
  Product1/1 -> Sum/1
  Fcn1/1 -> Product/2, Product1/2
  Integrator/1 -> Product/1, Out1/1
  In1/1 -> Product1/1
  In2/1 -> Fcn1/1

== system NeuronSizeActivity/Small  NewNeuron/Ion Channel11/Inertial Link (H1) ==
  In1 : Inport
  In2 : Inport  Port=2
  Fcn1 : Fcn  Expr=1/u
  Integrator : Integrator
  Product : Product  SaturateOnIntegerOverflow=on  RndMeth=Zero  InputSameDT=on  OutDataTypeStr=Inherit: Same as first input
  Product1 : Product  SaturateOnIntegerOverflow=on  RndMeth=Zero  InputSameDT=on  OutDataTypeStr=Inherit: Same as first input
  Sum : Sum  Inputs=+-  SaturateOnIntegerOverflow=on  InputSameDT=on  OutDataTypeStr=Inherit: Same as first input
  Out1 : Outport  InitialOutput=0
  wires:
  Sum/1 -> Integrator/1
  Product/1 -> Sum/2
  Product1/1 -> Sum/1
  Fcn1/1 -> Product/2, Product1/2
  Integrator/1 -> Product/1, Out1/1
  In1/1 -> Product1/1
  In2/1 -> Fcn1/1

== system NeuronSizeActivity/Small  NewNeuron1/Ion Channel11/Inertial Link (H1) ==
  In1 : Inport
  In2 : Inport  Port=2
  Fcn1 : Fcn  Expr=1/u
  Integrator : Integrator
  Product : Product  SaturateOnIntegerOverflow=on  RndMeth=Zero  InputSameDT=on  OutDataTypeStr=Inherit: Same as first input
  Product1 : Product  SaturateOnIntegerOverflow=on  RndMeth=Zero  InputSameDT=on  OutDataTypeStr=Inherit: Same as first input
  Sum : Sum  Inputs=+-  SaturateOnIntegerOverflow=on  InputSameDT=on  OutDataTypeStr=Inherit: Same as first input
  Out1 : Outport  InitialOutput=0
  wires:
  Sum/1 -> Integrator/1
  Product/1 -> Sum/2
  Product1/1 -> Sum/1
  Fcn1/1 -> Product/2, Product1/2
  Integrator/1 -> Product/1, Out1/1
  In1/1 -> Product1/1
  In2/1 -> Fcn1/1

== system NeuronSizeActivity/Small  NewNeuron2/Ion Channel11/Inertial Link (H1) ==
  In1 : Inport
  In2 : Inport  Port=2
  Fcn1 : Fcn  Expr=1/u
  Integrator : Integrator
  Product : Product  SaturateOnIntegerOverflow=on  RndMeth=Zero  InputSameDT=on  OutDataTypeStr=Inherit: Same as first input
  Product1 : Product  SaturateOnIntegerOverflow=on  RndMeth=Zero  InputSameDT=on  OutDataTypeStr=Inherit: Same as first input
  Sum : Sum  Inputs=+-  SaturateOnIntegerOverflow=on  InputSameDT=on  OutDataTypeStr=Inherit: Same as first input
  Out1 : Outport  InitialOutput=0
  wires:
  Sum/1 -> Integrator/1
  Product/1 -> Sum/2
  Product1/1 -> Sum/1
  Fcn1/1 -> Product/2, Product1/2
  Integrator/1 -> Product/1, Out1/1
  In1/1 -> Product1/1
  In2/1 -> Fcn1/1

== system NeuronSizeActivity/Small  NewNeuron3/Ion Channel11/Inertial Link (H1) ==
  In1 : Inport
  In2 : Inport  Port=2
  Fcn1 : Fcn  Expr=1/u
  Integrator : Integrator
  Product : Product  SaturateOnIntegerOverflow=on  RndMeth=Zero  InputSameDT=on  OutDataTypeStr=Inherit: Same as first input
  Product1 : Product  SaturateOnIntegerOverflow=on  RndMeth=Zero  InputSameDT=on  OutDataTypeStr=Inherit: Same as first input
  Sum : Sum  Inputs=+-  SaturateOnIntegerOverflow=on  InputSameDT=on  OutDataTypeStr=Inherit: Same as first input
  Out1 : Outport  InitialOutput=0
  wires:
  Sum/1 -> Integrator/1
  Product/1 -> Sum/2
  Product1/1 -> Sum/1
  Fcn1/1 -> Product/2, Product1/2
  Integrator/1 -> Product/1, Out1/1
  In1/1 -> Product1/1
  In2/1 -> Fcn1/1

== system NeuronSizeActivity/Small  NewNeuron4/Ion Channel11/Inertial Link (H1) ==
  In1 : Inport
  In2 : Inport  Port=2
  Fcn1 : Fcn  Expr=1/u
  Integrator : Integrator
  Product : Product  SaturateOnIntegerOverflow=on  RndMeth=Zero  InputSameDT=on  OutDataTypeStr=Inherit: Same as first input
  Product1 : Product  SaturateOnIntegerOverflow=on  RndMeth=Zero  InputSameDT=on  OutDataTypeStr=Inherit: Same as first input
  Sum : Sum  Inputs=+-  SaturateOnIntegerOverflow=on  InputSameDT=on  OutDataTypeStr=Inherit: Same as first input
  Out1 : Outport  InitialOutput=0
  wires:
  Sum/1 -> Integrator/1
  Product/1 -> Sum/2
  Product1/1 -> Sum/1
  Fcn1/1 -> Product/2, Product1/2
  Integrator/1 -> Product/1, Out1/1
  In1/1 -> Product1/1
  In2/1 -> Fcn1/1

== system NeuronSizeActivity/Small  NewNeuron5/Ion Channel11/Inertial Link (H1) ==
  In1 : Inport
  In2 : Inport  Port=2
  Fcn1 : Fcn  Expr=1/u
  Integrator : Integrator
  Product : Product  SaturateOnIntegerOverflow=on  RndMeth=Zero  InputSameDT=on  OutDataTypeStr=Inherit: Same as first input
  Product1 : Product  SaturateOnIntegerOverflow=on  RndMeth=Zero  InputSameDT=on  OutDataTypeStr=Inherit: Same as first input
  Sum : Sum  Inputs=+-  SaturateOnIntegerOverflow=on  InputSameDT=on  OutDataTypeStr=Inherit: Same as first input
  Out1 : Outport  InitialOutput=0
  wires:
  Sum/1 -> Integrator/1
  Product/1 -> Sum/2
  Product1/1 -> Sum/1
  Fcn1/1 -> Product/2, Product1/2
  Integrator/1 -> Product/1, Out1/1
  In1/1 -> Product1/1
  In2/1 -> Fcn1/1
